simulink model "question6_2_simulink"  (R2025b)
settings: Solver=ode45  StartTime=0.0  StopTime=5  RelTol=1e-3
settings Model: Creator=artes  LastModifiedBy=artes

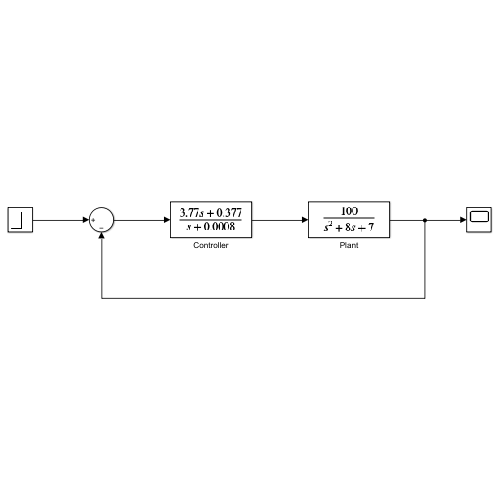
[thumbnail: Simulink's stored preview of the top-level diagram]
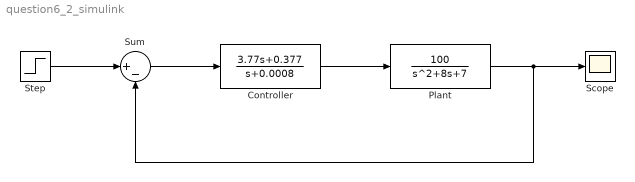
== system question6_2_simulink ==
  Controller : TransferFcn  Numerator=[3.77 0.377]  Denominator=[1 0.0008]
  Plant : TransferFcn  Numerator=[100]  Denominator=[1 8 7]
  Scope : Scope
  Step : Step  Time=0  SampleTime=0
  Sum : Sum  Inputs=|+-
  wires:
  Step/1 -> Sum/1
  Sum/1 -> Controller/1
  Controller/1 -> Plant/1
  Plant/1 -> Scope/1, Sum/2
